simulink model "USV1_Trajectory_Tracking_PID_Fuzzy4_BachelorThesis"  (R2018a)
settings: Solver=FixedStepAuto  StartTime=0.0  StopTime=400  FixedStep=1e-2  RelTol=1e-2
values from neighbouring files (symbols this model uses):
  A = [A_CAME; A_IKE; A_CLME]    [Prototype.m]    (also in USV1_PID_Fuzzy_Parameters.m = Mass\(-Coriolis - D_l))
  B = [B_CAME; B_IKE; B_CLME]    [Prototype.m]    (also in USV1_PID_Fuzzy_Parameters.m = Mass\F)
  C = eye(9)    [Prototype.m]    (also in USV1_PID_Fuzzy_Parameters.m = eye(4))
  D = zeros(9,4)    [Prototype.m]    (also in USV1_PID_Fuzzy_Parameters.m = [ 0  0  0 ;       0  0  0 ;       0  0  0 ;       0  0  0 ])
  Width = 1.83    [USV1_PID_Fuzzy_Parameters.m]
libraries: simulink x3, fuzblock x2
settings Model: Creator=admin  LastModifiedBy=MyPC
settings SolverCC: ZeroCrossControl=DisableAll  ZeroCrossAlgorithm=Adaptive
settings DebuggingCC: MaxConsecutiveZCsMsg=none  MaskedZcDiagnostic=none

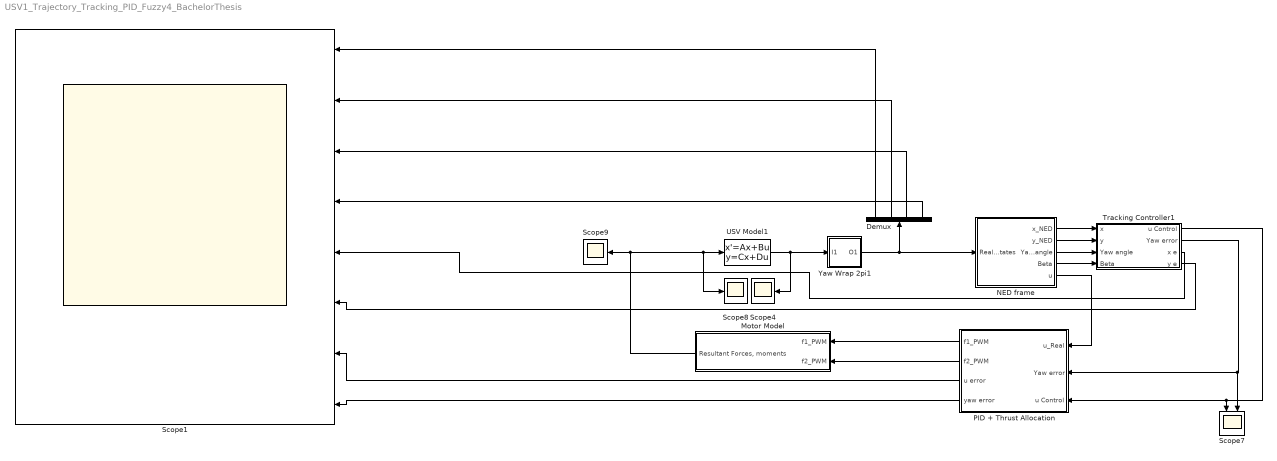
== system USV1_Trajectory_Tracking_PID_Fuzzy4_BachelorThesis ==
  Demux : Demux
  Motor Model : Subsystem
  NED frame : Subsystem
  PID + Thrust Allocation : Subsystem
  Scope1 : Scope  NumInputPorts=8
  Scope4 : Scope
  Scope7 : Scope  NumInputPorts=2
  Scope8 : Scope
  Scope9 : Scope
  Tracking Controller1 : Subsystem
  USV Model1 : StateSpace  A=A  B=B  C=C  D=D  InitialCondition=[0 0 0 pi/4]
  Yaw Wrap 2pi1 : Subsystem
  wires:
  Tracking Controller1/2(Yaw error) -> PID + Thrust Allocation/2(Yaw error), Scope7/2
  USV Model1/1 -> Scope4/1, Yaw Wrap 2pi1/1(I1)
  PID + Thrust Allocation/2(f2_PWM) -> Motor Model/2(f2_PWM)
  Motor Model/1("Resultant Forces, moments") -> Scope9/1, Scope8/1, USV Model1/1
  NED frame/1(x_NED) -> Tracking Controller1/1(x)
  Yaw Wrap 2pi1/1(O1) -> NED frame/1(Real states), Demux/1
  NED frame/2(y_NED) -> Tracking Controller1/2(y)
  NED frame/5(u) -> PID + Thrust Allocation/1(u_Real)
  Tracking Controller1/1(u Control) -> PID + Thrust Allocation/3(u Control), Scope7/1
  NED frame/3(Yaw_angle) -> Tracking Controller1/3(Yaw angle)
  PID + Thrust Allocation/1(f1_PWM) -> Motor Model/1(f1_PWM)
  NED frame/4(Beta) -> Tracking Controller1/4(Beta)
  Tracking Controller1/3(x e) -> Scope1/5
  Tracking Controller1/4(y e) -> Scope1/6
  PID + Thrust Allocation/3(u error) -> Scope1/7
  PID + Thrust Allocation/4(yaw error) -> Scope1/8
  Demux/1 -> Scope1/1
  Demux/2 -> Scope1/2
  Demux/3 -> Scope1/3
  Demux/4 -> Scope1/4

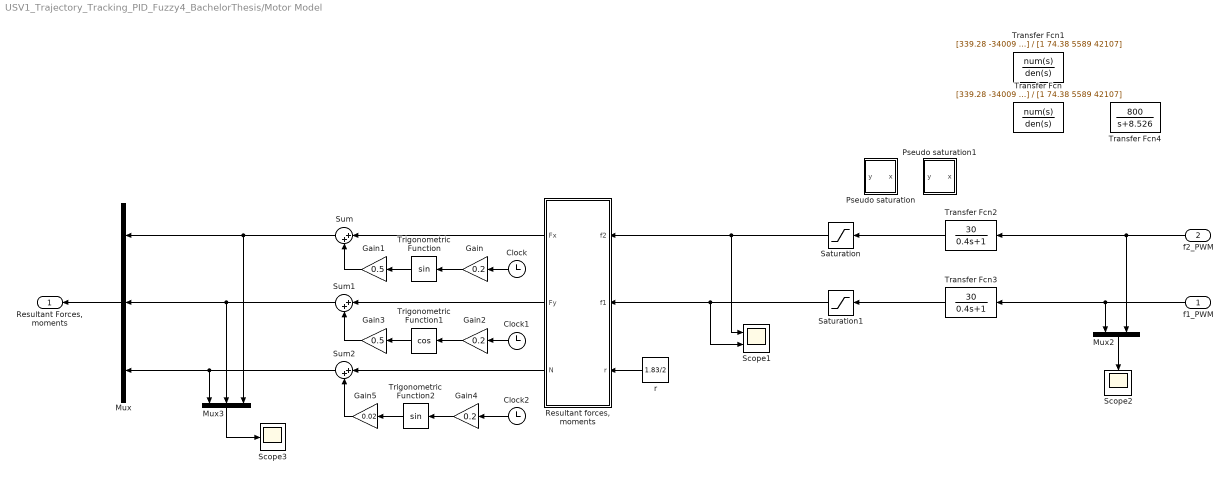
== system USV1_Trajectory_Tracking_PID_Fuzzy4_BachelorThesis/Motor Model ==
  f1_PWM : Inport
  f2_PWM : Inport  Port=2
  Clock : Clock
  Clock1 : Clock
  Clock2 : Clock
  Gain : Gain  Gain=0.2
  Gain1 : Gain  Gain=0.5
  Gain2 : Gain  Gain=0.2
  Gain3 : Gain  Gain=0.5
  Gain4 : Gain  Gain=0.2
  Gain5 : Gain  Gain=0.02
  Mux : Mux  Inputs=3
  Mux2 : Mux  Inputs=2
  Mux3 : Mux  Inputs=3
  Pseudo saturation : MATLAB Function  TreatAsAtomicUnit=on
  Pseudo saturation1 : MATLAB Function  TreatAsAtomicUnit=on
  "Resultant forces, moments" : MATLAB Function  TreatAsAtomicUnit=on
  Saturation : Saturate  UpperLimit=150  LowerLimit=0
  Saturation1 : Saturate  UpperLimit=150  LowerLimit=0
  Scope1 : Scope  NumInputPorts=2
  Scope2 : Scope
  Scope3 : Scope
  Sum : Sum  Inputs=|++
  Sum1 : Sum  Inputs=|++
  Sum2 : Sum  Inputs=|++
  Transfer Fcn : TransferFcn  Numerator=[339.28 -34009 3945100]  Denominator=[1 74.38 5589 42107]
  Transfer Fcn1 : TransferFcn  Numerator=[339.28 -34009 3945100]  Denominator=[1 74.38 5589 42107]
  Transfer Fcn2 : TransferFcn  Numerator=[30]  Denominator=[0.4 1]
  Transfer Fcn3 : TransferFcn  Numerator=[30]  Denominator=[0.4 1]
  Transfer Fcn4 : TransferFcn  Numerator=800  Denominator=[1 8.526]
  Trigonometric Function : Trigonometry
  Trigonometric Function1 : Trigonometry  Operator=cos
  Trigonometric Function2 : Trigonometry
  r : Constant  Value=1.83/2
  "Resultant Forces, moments" : Outport
  wires:
  Mux2/1 -> Scope2/1
  Saturation/1 -> Scope1/1, "Resultant forces, moments"/1(f2)
  r/1 -> "Resultant forces, moments"/3(r)
  Saturation1/1 -> Scope1/2, "Resultant forces, moments"/2(f1)
  Mux/1 -> "Resultant Forces, moments"/1
  Mux3/1 -> Scope3/1
  f1_PWM/1 -> Transfer Fcn3/1, Mux2/1
  f2_PWM/1 -> Transfer Fcn2/1, Mux2/2
  "Resultant forces, moments"/1(Fx) -> Sum/1
  Sum/1 -> Mux3/3, Mux/1
  "Resultant forces, moments"/2(Fy) -> Sum1/1
  Sum1/1 -> Mux3/2, Mux/2
  "Resultant forces, moments"/3(N) -> Sum2/1
  Sum2/1 -> Mux3/1, Mux/3
  Trigonometric Function/1 -> Gain1/1
  Clock/1 -> Gain/1
  Gain/1 -> Trigonometric Function/1
  Gain1/1 -> Sum/2
  Gain2/1 -> Trigonometric Function1/1
  Clock1/1 -> Gain2/1
  Trigonometric Function1/1 -> Gain3/1
  Gain3/1 -> Sum1/2
  Gain4/1 -> Trigonometric Function2/1
  Trigonometric Function2/1 -> Gain5/1
  Clock2/1 -> Gain4/1
  Gain5/1 -> Sum2/2
  Transfer Fcn2/1 -> Saturation/1
  Transfer Fcn3/1 -> Saturation1/1

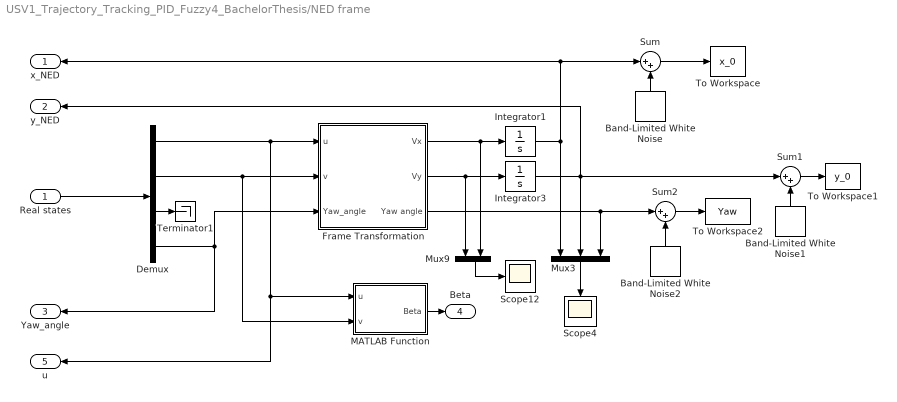
== system USV1_Trajectory_Tracking_PID_Fuzzy4_BachelorThesis/NED frame ==
  Real states : Inport
  Band-Limited White Noise : simulink/Sources/Band-Limited White Noise  Cov=0  Ts=0.1  seed=[23341]
  Band-Limited White Noise1 : simulink/Sources/Band-Limited White Noise  Cov=0  Ts=0.1  seed=[23341]
  Band-Limited White Noise2 : simulink/Sources/Band-Limited White Noise  Cov=0  Ts=0.1  seed=[23341]
  Demux : Demux
  Frame Transformation : Subsystem
  Integrator1 : Integrator
  Integrator3 : Integrator
  MATLAB Function : MATLAB Function  TreatAsAtomicUnit=on
  Mux3 : Mux  Inputs=3
  Mux9 : Mux  Inputs=2
  Scope12 : Scope
  Scope4 : Scope
  Sum : Sum  Inputs=|++
  Sum1 : Sum  Inputs=|++
  Sum2 : Sum  Inputs=|++
  Terminator1 : Terminator
  To Workspace : ToWorkspace  VariableName=x_0  SampleTime=-1
  To Workspace1 : ToWorkspace  VariableName=y_0  SampleTime=-1
  To Workspace2 : ToWorkspace  VariableName=Yaw  SampleTime=-1
  x_NED : Outport
  y_NED : Outport  Port=2
  Yaw_angle : Outport  Port=3
  Beta : Outport  Port=4
  u : Outport  Port=5
  wires:
  Demux/2 -> MATLAB Function/2(v), Frame Transformation/2(v)
  Frame Transformation/1(Vx) -> Integrator1/1, Mux9/2
  Mux9/1 -> Scope12/1
  Demux/3 -> Terminator1/1
  Integrator3/1 -> Sum1/1, y_NED/1, Mux3/2
  Frame Transformation/3(Yaw angle) -> Sum2/1, Mux3/3
  Mux3/1 -> Scope4/1
  Demux/1 -> MATLAB Function/1(u), u/1, Frame Transformation/1(u)
  Frame Transformation/2(Vy) -> Integrator3/1, Mux9/1
  Demux/4 -> Yaw_angle/1, Frame Transformation/3(Yaw_angle)
  Real states/1 -> Demux/1
  MATLAB Function/1(Beta) -> Beta/1
  Integrator1/1 -> Sum/1, x_NED/1, Mux3/1
  Sum/1 -> To Workspace/1
  Band-Limited White Noise/1 -> Sum/2
  Band-Limited White Noise1/1 -> Sum1/2
  Sum1/1 -> To Workspace1/1
  Sum2/1 -> To Workspace2/1
  Band-Limited White Noise2/1 -> Sum2/2

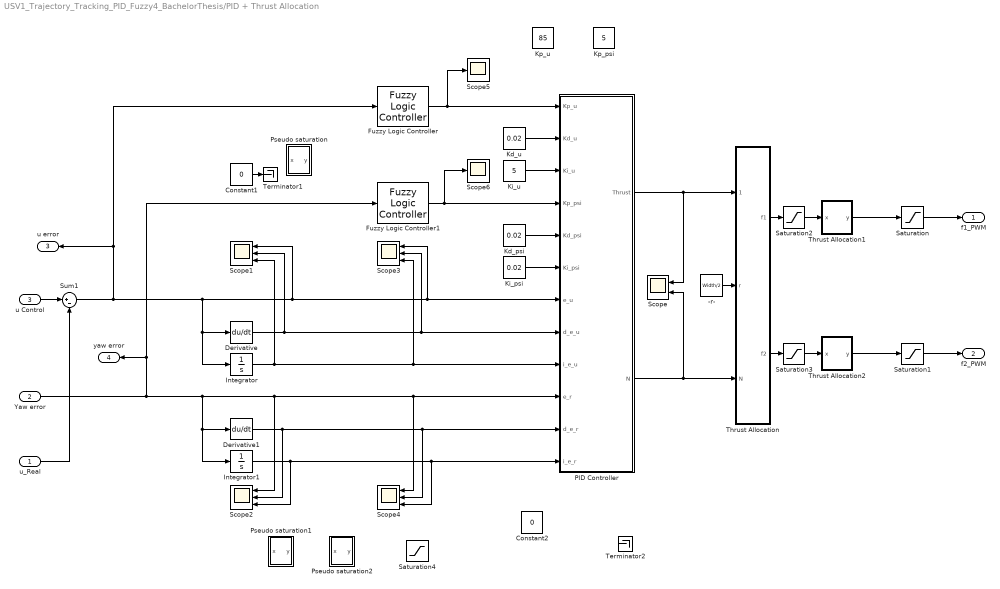
== system USV1_Trajectory_Tracking_PID_Fuzzy4_BachelorThesis/PID + Thrust Allocation ==
  u_Real : Inport
  Yaw error : Inport  Port=2
  u Control : Inport  Port=3
  "-r- " : Constant  Value=Width/2
  Constant1 : Constant  Value=0
  Constant2 : Constant  Value=0
  Derivative : Derivative
  Derivative1 : Derivative
  Fuzzy Logic Controller : fuzblock/Fuzzy Logic  Controller  FIS='FuzzyTrajectoryTrackingSugeno10.fis'  OutputSampleNumber=101  DataType=double  FuzzifiedInputs=off  RuleFiringStrengths=off  RuleOutputs=off  AggregatedOutputs=off  SimulateUsing=Interpreted execution  OutOfRangeInputValueMessage=warning  NoRuleFiredMessage=warning  EmptyOutputFuzzySetMessage=warning
  Fuzzy Logic Controller1 : fuzblock/Fuzzy Logic  Controller  FIS='FuzzyTrajectoryTrackingSugenoYaw6.fis'  OutputSampleNumber=101  DataType=double  FuzzifiedInputs=off  RuleFiringStrengths=off  RuleOutputs=off  AggregatedOutputs=off  SimulateUsing=Interpreted execution  OutOfRangeInputValueMessage=warning  NoRuleFiredMessage=warning  EmptyOutputFuzzySetMessage=warning
  Integrator : Integrator
  Integrator1 : Integrator
  Kd_psi : Constant  Value=0.02
  "Kd_u " : Constant  Value=0.02
  Ki_psi : Constant  Value=0.02
  Ki_u : Constant  Value=5
  Kp_psi : Constant  Value=5
  Kp_u : Constant  Value=85
  PID Controller : MATLAB Function  TreatAsAtomicUnit=on
  Pseudo saturation : MATLAB Function  TreatAsAtomicUnit=on
  Pseudo saturation1 : MATLAB Function  TreatAsAtomicUnit=on
  Pseudo saturation2 : MATLAB Function  TreatAsAtomicUnit=on
  Saturation : Saturate  UpperLimit=5  LowerLimit=0  LinearizeAsGain=off
  Saturation1 : Saturate  UpperLimit=5  LowerLimit=0  LinearizeAsGain=off
  Saturation2 : Saturate  UpperLimit=inf  LowerLimit=0  LinearizeAsGain=off
  Saturation3 : Saturate  UpperLimit=inf  LowerLimit=0  LinearizeAsGain=off
  Saturation4 : Saturate  UpperLimit=5  LowerLimit=-5
  Scope : Scope  NumInputPorts=2
  Scope{1..4} (4 alike) : Scope  NumInputPorts=3
  Scope5 : Scope
  Scope6 : Scope
  Sum1 : Sum  Inputs=|+-
  Terminator1 : Terminator
  Terminator2 : Terminator
  Thrust Allocation : MATLAB Function  TreatAsAtomicUnit=on
  Thrust Allocation1 : MATLAB Function  TreatAsAtomicUnit=on
  Thrust Allocation2 : MATLAB Function  TreatAsAtomicUnit=on
  f1_PWM : Outport
  f2_PWM : Outport  Port=2
  u error : Outport  Port=3
  yaw error : Outport  Port=4
  wires:
  Thrust Allocation/2(f2) -> Saturation3/1
  Thrust Allocation/1(f1) -> Saturation2/1
  "-r- "/1 -> Thrust Allocation/2(r)
  PID Controller/1(Thrust) -> Scope/1, Thrust Allocation/1(Thrust)
  PID Controller/2(N) -> Scope/2, Thrust Allocation/3(N)
  "Kd_u "/1 -> PID Controller/2(Kd_u)
  Derivative/1 -> Scope3/2, PID Controller/8(d_e_u), Scope1/2
  Ki_u/1 -> PID Controller/3(Ki_u)
  u_Real/1 -> Sum1/2
  u Control/1 -> Sum1/1
  Ki_psi/1 -> PID Controller/6(Ki_psi)
  Kd_psi/1 -> PID Controller/5(Kd_psi)
  Sum1/1 -> Fuzzy Logic Controller/1, u error/1, PID Controller/7(e_u), Scope3/1, Scope1/1, Derivative/1, Integrator/1
  Integrator/1 -> Scope3/3, PID Controller/9(i_e_u), Scope1/3
  Integrator1/1 -> Scope4/3, PID Controller/12(i_e_r), Scope2/3
  Derivative1/1 -> Scope4/2, PID Controller/11(d_e_r), Scope2/2
  Thrust Allocation1/1(y) -> Saturation/1
  Thrust Allocation2/1(y) -> Saturation1/1
  Constant1/1 -> Terminator1/1
  Saturation/1 -> f1_PWM/1
  Saturation1/1 -> f2_PWM/1
  Yaw error/1 -> Fuzzy Logic Controller1/1, yaw error/1, Scope4/1, PID Controller/10(e_r), Scope2/1, Integrator1/1, Derivative1/1
  Fuzzy Logic Controller/1 -> Scope5/1, PID Controller/1(Kp_u)
  Fuzzy Logic Controller1/1 -> PID Controller/4(Kp_psi), Scope6/1
  Saturation2/1 -> Thrust Allocation1/1(x)
  Saturation3/1 -> Thrust Allocation2/1(x)

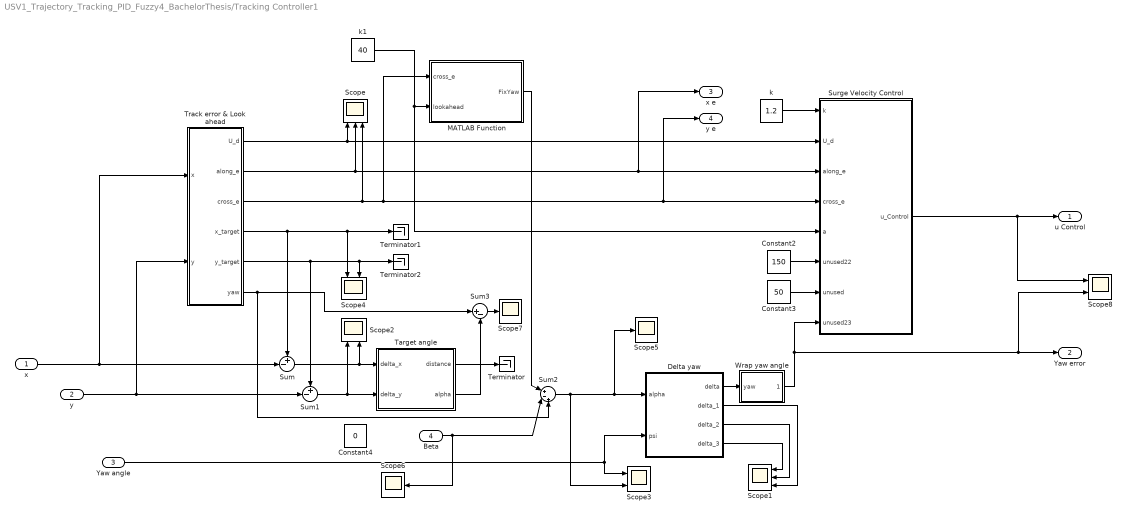
== system USV1_Trajectory_Tracking_PID_Fuzzy4_BachelorThesis/Tracking Controller1 ==
  x : Inport
  y : Inport  Port=2
  Yaw angle : Inport  Port=3
  Beta : Inport  Port=4
  Constant2 : Constant  Value=150
  Constant3 : Constant  Value=50
  Constant4 : Constant  Value=0
  Delta yaw : MATLAB Function  TreatAsAtomicUnit=on
  MATLAB Function : MATLAB Function  TreatAsAtomicUnit=on
  Scope : Scope  NumInputPorts=3
  Scope1 : Scope  NumInputPorts=3
  Scope{2..4,8} (4 alike) : Scope  NumInputPorts=2
  Scope5 : Scope
  Scope6 : Scope
  Scope7 : Scope
  Sum : Sum  Inputs=+-|
  Sum1 : Sum  Inputs=+-|
  Sum2 : Sum  Inputs=|+-+
  Sum3 : Sum  Inputs=|+-
  Surge Velocity Control : MATLAB Function  TreatAsAtomicUnit=on
  Target angle : MATLAB Function  TreatAsAtomicUnit=on
  Terminator : Terminator
  Terminator1 : Terminator
  Terminator2 : Terminator
  Track error & Look ahead : Subsystem
  Wrap yaw angle : MATLAB Function  TreatAsAtomicUnit=on
  k : Constant  Value=1.2
  k1 : Constant  Value=40
  u Control : Outport
  Yaw error : Outport  Port=2
  x e : Outport  Port=3
  y e : Outport  Port=4
  wires:
  Sum1/1 -> Scope2/1, Target angle/2(delta_y)
  y/1 -> Sum1/2, Track error & Look ahead/2(y)
  x/1 -> Sum/2, Track error & Look ahead/1(x)
  Surge Velocity Control/1(u_Control) -> Scope8/1, u Control/1
  Yaw angle/1 -> Delta yaw/2(psi), Scope3/1
  Track error & Look ahead/4(x_target) -> Sum/1, Terminator1/1, Scope4/1
  Track error & Look ahead/5(y_target) -> Sum1/1, Terminator2/1, Scope4/2
  Target angle/1(distance) -> Terminator/1
  Track error & Look ahead/1(U_d) -> Scope/1, Surge Velocity Control/2(U_d)
  k/1 -> Surge Velocity Control/1(k)
  Constant3/1 -> Surge Velocity Control/7(unused)
  Constant2/1 -> Surge Velocity Control/6(unused22)
  Track error & Look ahead/3(cross_e) -> Scope/3, y e/1, Surge Velocity Control/4(cross_e), MATLAB Function/1(cross_e)
  Delta yaw/4(delta_3) -> Scope1/1
  Delta yaw/3(delta_2) -> Scope1/2
  Delta yaw/2(delta_1) -> Scope1/3
  Sum2/1 -> Scope3/2, Scope5/1, Delta yaw/1(alpha)
  Beta/1 -> Scope6/1, Sum2/2
  Sum/1 -> Scope2/2, Target angle/1(delta_x)
  Track error & Look ahead/6(yaw) -> Sum2/3, Sum3/1
  Sum3/1 -> Scope7/1
  MATLAB Function/1(FixYaw) -> Sum2/1
  Delta yaw/1(delta) -> Wrap yaw angle/1(yaw)
  Wrap yaw angle/1(yaw_2pi) -> Yaw error/1, Scope8/2, Surge Velocity Control/8(unused23)
  Track error & Look ahead/2(along_e) -> Scope/2, x e/1, Surge Velocity Control/3(along_e)
  k1/1 -> Surge Velocity Control/5(a), MATLAB Function/2(lookahead)
  Target angle/2(alpha) -> Sum3/2

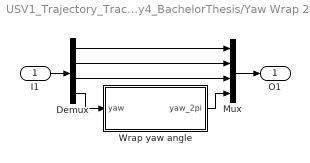
== system USV1_Trajectory_Tracking_PID_Fuzzy4_BachelorThesis/Yaw Wrap 2pi1 ==
  I1 : Inport
  Demux : Demux
  Mux : Mux
  Wrap yaw angle : MATLAB Function  TreatAsAtomicUnit=on
  O1 : Outport
  wires:
  Demux/1 -> Mux/1
  Demux/3 -> Mux/3
  I1/1 -> Demux/1
  Wrap yaw angle/1(yaw_2pi) -> Mux/4
  Mux/1 -> O1/1
  Demux/4 -> Wrap yaw angle/1(yaw)
  Demux/2 -> Mux/2

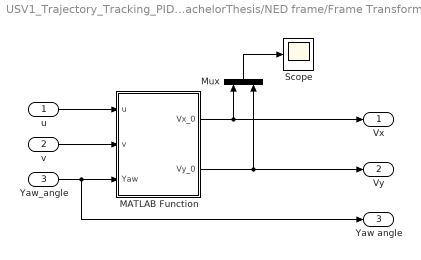
== system USV1_Trajectory_Tracking_PID_Fuzzy4_BachelorThesis/NED frame/Frame Transformation ==
  u : Inport
  v : Inport  Port=2
  Yaw_angle : Inport  Port=3
  MATLAB Function : MATLAB Function  TreatAsAtomicUnit=on
  Mux : Mux  Inputs=2
  Scope : Scope
  Vx : Outport
  Vy : Outport  Port=2
  Yaw angle : Outport  Port=3
  wires:
  v/1 -> MATLAB Function/2(v)
  MATLAB Function/1(Vx_0) -> Vx/1, Mux/1
  u/1 -> MATLAB Function/1(u)
  MATLAB Function/2(Vy_0) -> Vy/1, Mux/2
  Yaw_angle/1 -> MATLAB Function/3(Yaw), Yaw angle/1
  Mux/1 -> Scope/1

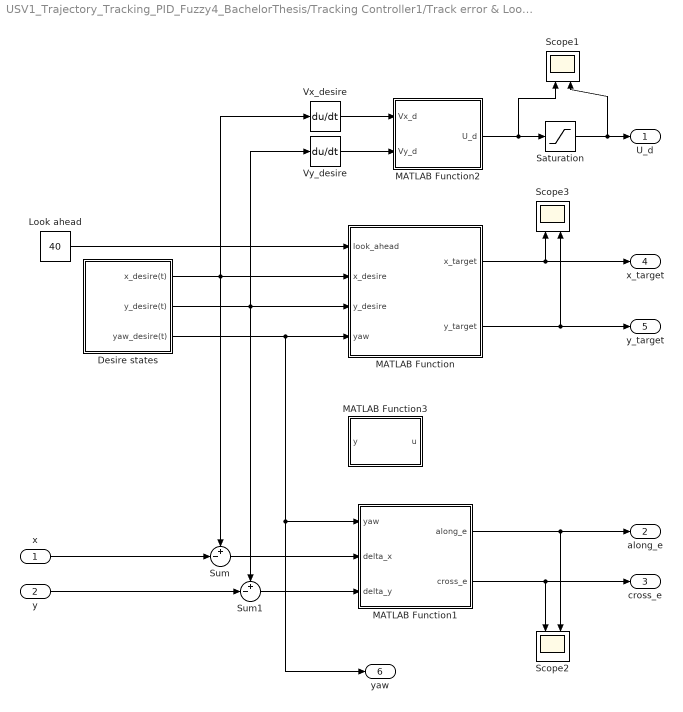
== system USV1_Trajectory_Tracking_PID_Fuzzy4_BachelorThesis/Tracking Controller1/Track error & Look ahead ==
  x : Inport
  y : Inport  Port=2
  Desire states : Subsystem
  Look ahead : Constant  Value=40
  MATLAB Function : MATLAB Function  TreatAsAtomicUnit=on
  MATLAB Function1 : MATLAB Function  TreatAsAtomicUnit=on
  MATLAB Function2 : MATLAB Function  TreatAsAtomicUnit=on
  MATLAB Function3 : MATLAB Function  TreatAsAtomicUnit=on
  Saturation : Saturate  UpperLimit=5  LowerLimit=-0.1
  Scope1 : Scope  NumInputPorts=2
  Scope2 : Scope  NumInputPorts=2
  Scope3 : Scope  NumInputPorts=2
  Sum : Sum  Inputs=+-|
  Sum1 : Sum  Inputs=+-|
  Vx_desire : Derivative
  Vy_desire : Derivative
  U_d : Outport
  along_e : Outport  Port=2
  cross_e : Outport  Port=3
  x_target : Outport  Port=4
  y_target : Outport  Port=5
  yaw : Outport  Port=6
  wires:
  Desire states/3(yaw_desire(t)) -> yaw/1, MATLAB Function1/1(yaw), MATLAB Function/4(yaw)
  Desire states/1(x_desire(t)) -> Vx_desire/1, Sum/1, MATLAB Function/2(x_desire)
  Desire states/2(y_desire(t)) -> Vy_desire/1, MATLAB Function/3(y_desire), Sum1/1
  Look ahead/1 -> MATLAB Function/1(look_ahead)
  MATLAB Function/1(x_target) -> Scope3/1, x_target/1
  MATLAB Function/2(y_target) -> Scope3/2, y_target/1
  x/1 -> Sum/2
  y/1 -> Sum1/2
  Sum1/1 -> MATLAB Function1/3(delta_y)
  Sum/1 -> MATLAB Function1/2(delta_x)
  Vx_desire/1 -> MATLAB Function2/1(Vx_d)
  Vy_desire/1 -> MATLAB Function2/2(Vy_d)
  MATLAB Function2/1(U_d) -> Saturation/1, Scope1/1
  MATLAB Function1/1(along_e) -> along_e/1, Scope2/2
  MATLAB Function1/2(cross_e) -> cross_e/1, Scope2/1
  Saturation/1 -> U_d/1, Scope1/2

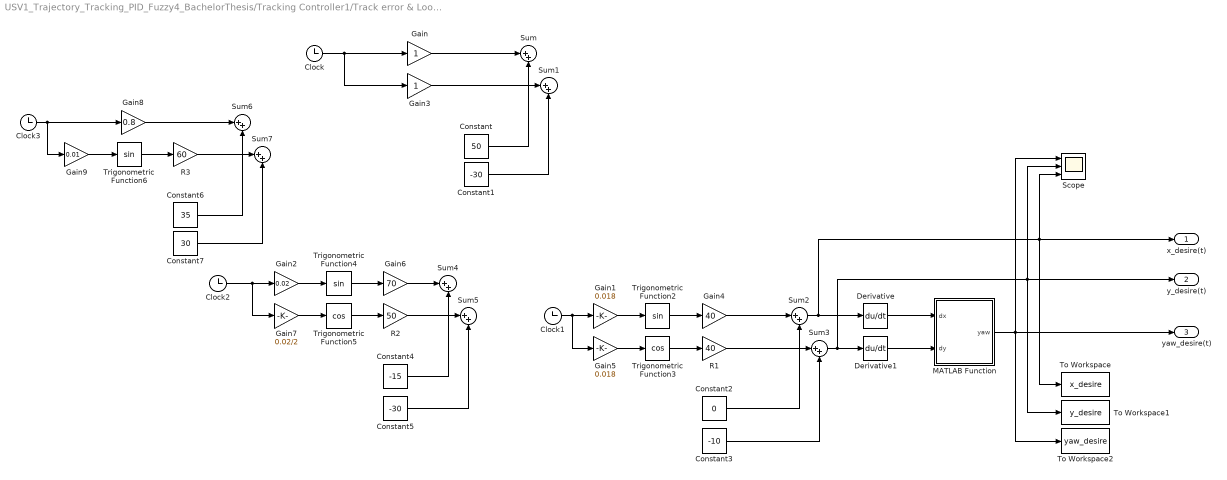
== system USV1_Trajectory_Tracking_PID_Fuzzy4_BachelorThesis/Tracking Controller1/Track error & Look ahead/Desire states ==
  Clock{,1..3} (4 alike) : Clock
  Constant : Constant  Value=50
  Constant1 : Constant  Value=-30
  Constant2 : Constant  Value=0
  Constant3 : Constant  Value=-10
  Constant4 : Constant  Value=-15
  Constant5 : Constant  Value=-30
  Constant6 : Constant  Value=35
  Constant7 : Constant  Value=30
  Derivative : Derivative
  Derivative1 : Derivative
  Gain : Gain
  Gain1 : Gain  Gain=0.018
  Gain2 : Gain  Gain=0.02
  Gain3 : Gain
  Gain4 : Gain  Gain=40
  Gain5 : Gain  Gain=0.018
  Gain6 : Gain  Gain=70
  Gain7 : Gain  Gain=0.02/2
  Gain8 : Gain  Gain=0.8
  Gain9 : Gain  Gain=0.01
  MATLAB Function : MATLAB Function  TreatAsAtomicUnit=on
  R1 : Gain  Gain=40
  R2 : Gain  Gain=50
  R3 : Gain  Gain=60
  Scope : Scope  NumInputPorts=3
  Sum{,1..7} (8 alike) : Sum  Inputs=|++
  To Workspace : ToWorkspace  VariableName=x_desire  SampleTime=-1
  To Workspace1 : ToWorkspace  VariableName=y_desire  SampleTime=-1
  To Workspace2 : ToWorkspace  VariableName=yaw_desire  SampleTime=-1
  Trigonometric Function2 : Trigonometry  OutputSignalType=real
  Trigonometric Function3 : Trigonometry  Operator=cos  OutputSignalType=real
  Trigonometric Function4 : Trigonometry  OutputSignalType=real
  Trigonometric Function5 : Trigonometry  Operator=cos  OutputSignalType=real
  Trigonometric Function6 : Trigonometry  OutputSignalType=real
  x_desire(t) : Outport
  y_desire(t) : Outport  Port=2
  yaw_desire(t) : Outport  Port=3
  wires:
  Derivative/1 -> MATLAB Function/1(dx)
  Derivative1/1 -> MATLAB Function/2(dy)
  MATLAB Function/1(yaw) -> To Workspace2/1, Scope/1, yaw_desire(t)/1
  Constant/1 -> Sum/2
  Constant1/1 -> Sum1/2
  Clock/1 -> Gain3/1, Gain/1
  Gain/1 -> Sum/1
  R1/1 -> Sum3/1
  Trigonometric Function3/1 -> R1/1
  Trigonometric Function2/1 -> Gain4/1
  Gain5/1 -> Trigonometric Function3/1
  Gain1/1 -> Trigonometric Function2/1
  Clock1/1 -> Gain1/1, Gain5/1
  Constant3/1 -> Sum3/2
  Constant2/1 -> Sum2/2
  Gain4/1 -> Sum2/1
  Gain7/1 -> Trigonometric Function5/1
  Trigonometric Function5/1 -> R2/1
  Constant4/1 -> Sum4/2
  Constant5/1 -> Sum5/2
  Clock2/1 -> Gain7/1, Gain2/1
  R2/1 -> Sum5/1
  Gain2/1 -> Trigonometric Function4/1
  Trigonometric Function4/1 -> Gain6/1
  Gain6/1 -> Sum4/1
  Constant7/1 -> Sum7/2
  Gain9/1 -> Trigonometric Function6/1
  Trigonometric Function6/1 -> R3/1
  R3/1 -> Sum7/1
  Gain8/1 -> Sum6/1
  Clock3/1 -> Gain9/1, Gain8/1
  Constant6/1 -> Sum6/2
  Gain3/1 -> Sum1/1
  Sum2/1 -> To Workspace/1, Scope/3, x_desire(t)/1, Derivative/1
  Sum3/1 -> To Workspace1/1, Scope/2, y_desire(t)/1, Derivative1/1

== matlab function USV1_Trajectory_Tracking_PID_Fuzzy4_BachelorThesis/PID + Thrust Allocation/Thrust Allocation1 ==
  data: x input; y output
function y = fcn(x)

%y = x/20;
%y=13.4*atanh(x/700)
%y = (x/25.5)^(1/1.1)
y=x/30;

== matlab function USV1_Trajectory_Tracking_PID_Fuzzy4_BachelorThesis/PID + Thrust Allocation/Thrust Allocation2 ==
  data: x input; y output
function y = fcn(x)

%y = x/20;
%y=13.4*atanh(x/420)
%y = (x/10)/sqrt((x^2/50^2)+2)
y=x/30;

== matlab function USV1_Trajectory_Tracking_PID_Fuzzy4_BachelorThesis/Motor Model/Pseudo saturation1 ==
  data: x input; y output
function y = fcn(x)

y = 410*tanh(x/20);

== matlab function USV1_Trajectory_Tracking_PID_Fuzzy4_BachelorThesis/Tracking Controller1/Track error & Look ahead/MATLAB Function3 ==
  data: u input; y output
function y = fcn(u)

y = u;

== matlab function USV1_Trajectory_Tracking_PID_Fuzzy4_BachelorThesis/Tracking Controller1/MATLAB Function ==
  data: cross_e input; FixYaw output; lookahead input
function FixYaw = fcn(cross_e,lookahead)
r = cross_e/(lookahead)
FixYaw = atan(r);

== matlab function USV1_Trajectory_Tracking_PID_Fuzzy4_BachelorThesis/Tracking Controller1/Wrap yaw angle ==
  data: yaw input; yaw_2pi output
function yaw_2pi = fcn(yaw)

yaw_2pi = atan2(sin(yaw),cos(yaw));

== matlab function USV1_Trajectory_Tracking_PID_Fuzzy4_BachelorThesis/Motor Model/Pseudo saturation ==
  data: x input; y output
function y = fcn(x)

y = 410*tanh(x/20);

== matlab function USV1_Trajectory_Tracking_PID_Fuzzy4_BachelorThesis/Motor Model/Resultant forces, moments ==
  data: f2 input; f1 input; r input; Fx output; Fy output; N output
function [Fx,Fy,N] = fcn(f2,f1,r)

Fx = f1 + f2;
Fy = 0;
N = f1*r - f2*r;

== matlab function USV1_Trajectory_Tracking_PID_Fuzzy4_BachelorThesis/NED frame/Frame Transformation/MATLAB Function ==
  data: u input; Vx_0 output; v input; Yaw input; Vy_0 output
function [Vx_0 , Vy_0 ] = fcn(u, v, Yaw)

Vx_0 =  cos(Yaw)*u - sin(Yaw)*v ;
Vy_0 =  sin(Yaw)*u + cos(Yaw)*v ;

== matlab function USV1_Trajectory_Tracking_PID_Fuzzy4_BachelorThesis/PID + Thrust Allocation/PID Controller ==
  data: Kp_u input; Thrust output; Kd_u input; Ki_u input; Kp_psi input; Kd_psi input; Ki_psi input; e_u input; d_e_u input; i_e_u input; e_r input; d_e_r input; N output; i_e_r input
function [Thrust, N] = fcn(Kp_u, Kd_u, Ki_u, Kp_psi, Kd_psi, Ki_psi, e_u,d_e_u,i_e_u, e_r,d_e_r,i_e_r)

Thrust = (e_u * Kp_u) + (d_e_u * Kd_u) + (i_e_u * Ki_u);
N = (e_r * Kp_psi) + (d_e_r * Kd_psi) + (i_e_r * Ki_psi);

== matlab function USV1_Trajectory_Tracking_PID_Fuzzy4_BachelorThesis/PID + Thrust Allocation/Pseudo saturation ==
  data: x input; y output
function y = fcn(x)

y = (4.5*x^2)/(x^2+5);

== matlab function USV1_Trajectory_Tracking_PID_Fuzzy4_BachelorThesis/PID + Thrust Allocation/Pseudo saturation1 ==
  data: x input; y output
function y = fcn(x)

y = (x*abs(x))/(x^2+0.3);

== matlab function USV1_Trajectory_Tracking_PID_Fuzzy4_BachelorThesis/PID + Thrust Allocation/Pseudo saturation2 ==
  data: x input; y output
function y = fcn(x)

y = (5*x*abs(x))/(x^2+4);

== matlab function USV1_Trajectory_Tracking_PID_Fuzzy4_BachelorThesis/PID + Thrust Allocation/Thrust Allocation ==
  data: Thrust input; r input; f1 output; N input; f2 output
function [f1,f2] = fcn(Thrust, r, N)

f1 = Thrust/2 + N/r;
f2 = Thrust/2 - N/r;

== matlab function USV1_Trajectory_Tracking_PID_Fuzzy4_BachelorThesis/Tracking Controller1/Delta yaw ==
  data: alpha input; delta output; psi input; delta_1 output; delta_2 output; delta_3 output
function [delta, delta_1, delta_2, delta_3] = fcn(alpha, psi)

delta_1 = alpha - psi;
delta_2 = delta_1 - 2*pi;
delta_3 = delta_1 + 2*pi;

delta = delta_1;

if abs(delta)>pi
    delta = delta_2;
end

== matlab function USV1_Trajectory_Tracking_PID_Fuzzy4_BachelorThesis/Tracking Controller1/Surge Velocity Control ==
  data: k input; U_d input; u_Control output; along_e input; cross_e input; a input; unused22 input; unused input; unused23 input
function u_Control =   fcn(k,U_d,along_e, cross_e, a, ~, ~, ~)

%k_yaw = 1/(32*(delta_psi^4) + 1);
%k_along = 0.2/(1/(along_e^2) + b);
%k_cross = 0.8+ ((0.2*cross_e^2)/(cross_e^2 + c));

%u_Control = (U_d*along_e + k*k_yaw*k_along);

%u_Control = U_d +k*k_along;

%u_Control = U_d + k*abs(along_e)/(sqrt(along_e^2+cross_e^2))

%u_Control = U_d * along_e/ (sqrt(along_e^2+cross_e^2)) 

%u_Control = (U_d - k*k_along);

%%%%u_Control = (U_d + k*along_e/(along_e^2+200))

%%%%%u_Control = U_d + k*along_e


%u_Control = (U_d - k*k_yaw*k_along)*k_cross;

%u_Control = (U_d+ k*along_e)*(sqrt((along_e+40)^2)+cross_e^2)/(abs(along_e+40))

%f_xe = (abs(along_e+40) + cross_e^2) / (sqrt((along_e+40)^2+cross_e^2));

%u_Control = (U_d* f_xe + k*along_e/f_xe)

%u_Control = (U_d + k*along_e)*sqrt(a^2+cross_e^2)/a

%%%%%%%u_Control = (U_d + k*along_e/(along_e^2 + 200))*sqrt(a^2+cross_e^2)/a;

%u_Control = (U_d * sqrt(a^2+cross_e^2) + k *along_e )/a

u_Control = (U_d + k*along_e/sqrt(a^2+along_e^2))*sqrt(a^2+cross_e^2)/a;

== matlab function USV1_Trajectory_Tracking_PID_Fuzzy4_BachelorThesis/Tracking Controller1/Target angle ==
  data: distance output; delta_x input; alpha output; delta_y input
function [distance,alpha] = fcn(delta_x, delta_y)

alpha = atan2(delta_y,delta_x);
distance = ((delta_x^2)+(delta_y^2))^0.5;

== matlab function USV1_Trajectory_Tracking_PID_Fuzzy4_BachelorThesis/Tracking Controller1/Track error & Look ahead/Desire states/MATLAB Function ==
  data: dx input; yaw output; dy input
function yaw = fcn(dx,dy)

yaw = atan2(dy,dx);

== matlab function USV1_Trajectory_Tracking_PID_Fuzzy4_BachelorThesis/Tracking Controller1/Track error & Look ahead/MATLAB Function ==
  data: look_ahead input; x_target output; x_desire input; y_desire input; yaw input; y_target output
function [x_target, y_target] = fcn(look_ahead, x_desire, y_desire, yaw)

x_target = x_desire + (look_ahead*cos(yaw));
y_target = y_desire + (look_ahead*sin(yaw));

== matlab function USV1_Trajectory_Tracking_PID_Fuzzy4_BachelorThesis/Tracking Controller1/Track error & Look ahead/MATLAB Function1 ==
  data: yaw input; along_e output; delta_x input; delta_y input; cross_e output
function [along_e, cross_e] = fcn(yaw, delta_x, delta_y)

along_e = (cos(yaw)*delta_x) + (sin(yaw)*delta_y);
cross_e = (-sin(yaw)*delta_x) + (cos(yaw)*delta_y);

== matlab function USV1_Trajectory_Tracking_PID_Fuzzy4_BachelorThesis/Tracking Controller1/Track error & Look ahead/MATLAB Function2 ==
  data: Vx_d input; U_d output; Vy_d input
function U_d = fcn(Vx_d, Vy_d)

U_d = ((Vx_d^2) + (Vy_d^2))^0.5;

== matlab function USV1_Trajectory_Tracking_PID_Fuzzy4_BachelorThesis/Yaw Wrap 2pi1/Wrap yaw angle ==
  data: yaw input; yaw_2pi output
function yaw_2pi = fcn(yaw)

yaw_2pi = atan2(sin(yaw),cos(yaw));

== matlab function USV1_Trajectory_Tracking_PID_Fuzzy4_BachelorThesis/NED frame/MATLAB Function ==
  data: u input; Beta output; v input
function Beta = fcn(u,v)

Beta = atan2(v,u);
